simulink model "FSM1"  (R2024a)
settings: Solver=VariableStepAuto  StartTime=0.0  StopTime=T  MaxStep=MaxStep  RelTol=RelTol
values from neighbouring files (symbols this model uses):
  J = 20    [Init.m]
  T = 10    [Init.m]
  x0 = 1    [Init.m]
libraries: HyEQ_Library x1
settings Model: Creator=venkat  LastModifiedBy=venkat

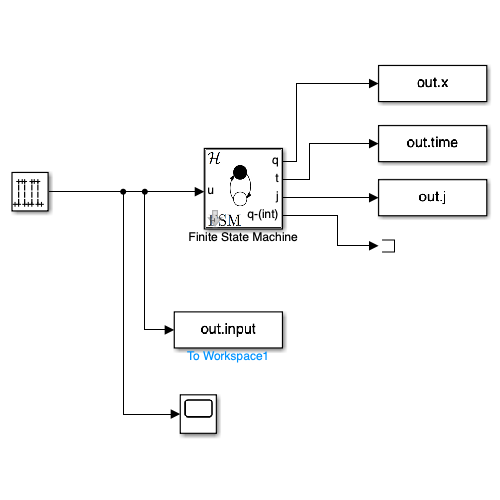
[thumbnail: Simulink's stored preview of the top-level diagram]
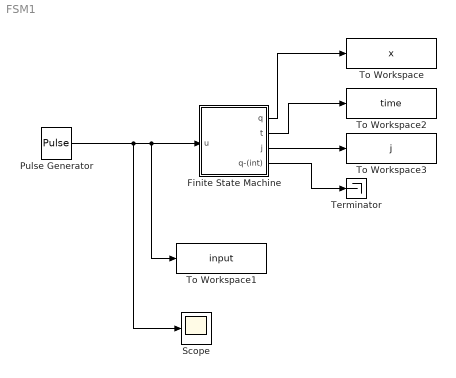
== system FSM1 ==
  Finite State Machine : Subsystem  LoadFcn=set_param(gcb,'LinkStatus','none')  mask(Finite State Machine (FSM)){q0=x0, input_dim=1, T=T, J=J}
      mask prompts: q0 "Initial state (column vector)"; input_dim "Input dimension (nonnegative integer)"; T "Flow Horizon (nonnegative real)"; J "Jump Horizon (nonnegative integer)"
      mask help:
      | To define the FSM:
      | 1. Select the block,
      | 2. "Look inside" the block: Either open the context menu and select Mask > Look Under Mask, or click the arrow in the bottom-left corner of the block.
      | 3. Edit the flow set C, jump set D, and jump map g.
      mask init:
      | state_dim = numel(q0);
      settings: CopyFcn=|
      | set_param(gcb,'LinkStatus','none'),
      | set_param(gcs, 'MaxStep', 'MaxStep', 'RelTol', 'RelTol','StopTime', 'T')
      mask Help: eval hybrid.internal.openHelp('CPS_finite_state_machine')
      mask TypeOptions T: Integrator System/T
      mask TypeOptions J: Integrator System/J
      mask DialogControl Control2 Prompt: CPS Components Documentation
      mask DialogControl Control2 Callback: hybrid.internal.openHelp('CPS_Components')
      mask DialogControl Container4 Prompt: Configuration
      mask Display:
      | image('FSM.jpg')
      | port_label('output', 1, 'q')
      | port_label('output', 2, 't')
      | port_label('output', 3, 'j')
      | port_label('output', 4, 'q-(int)')
      | port_label('input', 1, 'u')
  Pulse Generator : DiscretePulseGenerator  SampleTime=T
  Scope : Scope
  Terminator : Terminator
  To Workspace : ToWorkspace  VariableName=x  SampleTime=-1
  To Workspace1 : ToWorkspace  VariableName=input  SampleTime=-1
  To Workspace2 : ToWorkspace  VariableName=time  SampleTime=-1
  To Workspace3 : ToWorkspace  VariableName=j  SampleTime=-1
  wires:
  Pulse Generator/1 -> Scope/1, To Workspace1/1, Finite State Machine/1(u)
  Finite State Machine/1(q) -> To Workspace/1
  Finite State Machine/2(t) -> To Workspace2/1
  Finite State Machine/3(j) -> To Workspace3/1
  Finite State Machine/4(q-(int)) -> Terminator/1

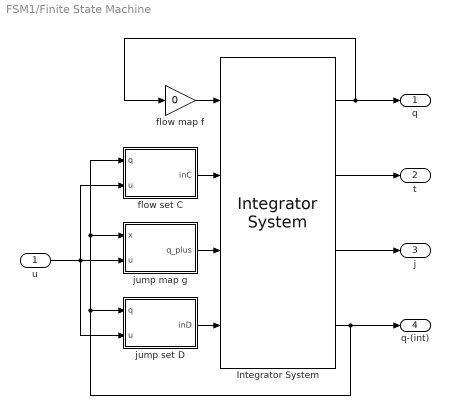
== system FSM1/Finite State Machine ==
  u : Inport  PortDimensions=input_dim
  Integrator System : HyEQ_Library/Other/Integrator System  Priority=2  T=T  J=J  x0=q0  rule=1
      settings: SourceProductName=Hybrid Equations Toolbox
  flow map f : Gain  Gain=0
  flow set C : MATLAB Function  TreatAsAtomicUnit=on
  jump map g : MATLAB Function  TreatAsAtomicUnit=on
  jump set D : MATLAB Function  TreatAsAtomicUnit=on
  q : Outport  PortDimensions=state_dim
  t : Outport  Port=2  PortDimensions=1
  j : Outport  Port=3  PortDimensions=1
  q-(int) : Outport  Port=4  PortDimensions=state_dim
  wires:
  jump map g/1(q_plus) -> Integrator System/3
  jump set D/1(inD) -> Integrator System/4
  u/1 -> jump map g/2(u), jump set D/2(u), flow set C/2(u)
  Integrator System/3 -> j/1
  Integrator System/2 -> t/1
  flow set C/1(inC) -> Integrator System/2
  Integrator System/1 -> q/1, flow map f/1
  Integrator System/4 -> q-(int)/1, flow set C/1(q), jump map g/1(x), jump set D/1(q)
  flow map f/1 -> Integrator System/1

== matlab function FSM1/Finite State Machine/jump map g ==
  data: x input size=state_dim; u input size=input_dim; q_plus output size=state_dim
function q_plus = g(x, u)
    % Jump map for finite state machine.
    q = x;
    q_plus = x;
    %truth table
    if (u(1) == 0) && ((q==1) || (q==2))
        q_plus = 1;
    elseif (u(1) == 0) && (q==3)
        q_plus = q;
    elseif (u(1) == 1) && (q==1)
        q_plus = 2;
    elseif (u(1) == 1) && ((q==2) || (q==3))
        q_plus = 3;
    end
end

== matlab function FSM1/Finite State Machine/jump set D ==
  data: q input size=state_dim; u input size=input_dim; inD output size=1
function inD  = D(q, u) 
    % Jump set indicator finite state machine.

    % Specify conditions for when the system should jump.
    inD = 1;
end

== matlab function FSM1/Finite State Machine/flow set C ==
  data: q input size=state_dim; u input size=input_dim; inC output size=1
function inC  = C(q, u) 
    % Flow set indicator function for finite state machine.
    
    % Specify conditions for when the system should flow.
    inC = 1;
end
